simulink model "EVX_Lap_Simulation"  (R2018b)
settings: Solver=FixedStepAuto  StartTime=0  StopTime=100  FixedStep=0.01  MinStep=0.001  RelTol=1e-3
undefined symbols (not defined in the file): Car, dist, DOD, initial_velocity, motorefficiency, motormaxtorque, motorspeedradps, R0model, theta_d, Track_Dist, velocity_dnew, VoltageDOD, x, y
libraries: simulink x4
(part 3 of 3)

== matlab function EVX_Lap_Simulation/EVX Vehicle Model/Vertical Dynamics/MATLAB Function3 ==
  data: V output; F input; zB input; D output; w input; kc input; kt input; ks input; kr input
function [V,D] = Initial_SS(F,zB,w,kc,kt,ks,kr)

% syms z_WFL z_WFR z_WRL z_WRR z_c thetay thetax_F thetax_R
% 
% eq_FL = F(1) + zB(1) * kt(1)...
% 	== z_WFL * (kt(1) + ks(1) + kr(1) + kr(3) + kr(5))...
% 	 + z_WFR * (-kr(1))...
%      + z_WRL * (-kr(2))...
%      + z_wRR * (-kr(5))...
%      + z_c * (-ks(1))...
%      + thetay * (w(1,1) * ks(1))...
%      + thetax_F * (-w(2,1) * ks(1))...
%      + thetax_R * (0);
%  
% eq_FR = F(2) + zB(2) * kt(2)...
% 	== z_WFL * (-kr(1))...
% 	 + z_WFR * (kt(2) + ks(2) + kr(1) + kr(4) + kr(6))...
%      + z_WRL * (-kr(6))...
%      + z_wRR * (-kr(4))...
%      + z_c * (-ks(2))...
%      + thetay * (w(1,2) * ks(2))...
%      + thetax_F * (-w(2,2) * ks(2))...
%      + thetax_R * (0);
% 
% eq_RL = F(3) + zB(3) * kt(3)...
% 	== z_WFL * (-kr(3))...
% 	 + z_WFR * (-kr(6))...
%      + z_WRL * (kt(3) + ks(3) + kr(2) + kr(3) + kr(6))...
%      + z_wRR * (-kr(2))...
%      + z_c * (-ks(3))...
%      + thetay * (w(1,3) * ks(3))...
%      + thetax_F * (0)...
%      + thetax_R * (-w(2,3) * ks(3));
%  
% eq_RR = F(4) + zB(4) * kt(4)...
% 	== z_WFL * (-kr(5))...
% 	 + z_WFR * (-kr(4))...
%      + z_WRL * (-kr(2))...
%      + z_wRR * (kt(4) + ks(4) + kr(2) + kr(4) + kr(5))...
%      + z_c * (-ks(4))...
%      + thetay * (w(1,4) * ks(4))...
%      + thetax_F * (0)...
%      + thetax_R * (-w(2,4) * ks(4));
%  
% eq_zc = F(5)...
%     == z_WFL * (-ks(1))...
%      + z_WFR * (-ks(2))...
%      + z_WRL * (-ks(3))...
%      + z_WRR * (-ks(4))...
%      + z_c * (ks(1) + ks(2) + ks(3) + ks(4))...
%      + thetay * (-W(1,1) * ks(1) - w(1,2) * ks(2) - w(1,3) * ks(3) - w(1,4) * ks(4))...
%      + thetax_F * (w(2,1) * ks(1) + w(2,2) * ks(2))...
%      + thetax_R * (w(2,3) * ks(3) + w(2,4) * ks(4));
%  
% eq_thetay = F(6)...
%     == z_WFL * (w(1,1) * ks(1))...
%      + z_WFR * (w(1,2) * ks(2))...
%      + z_WRL * (w(1,3) * ks(3))...
%      + z_WRR * (w(1,4) * ks(4))...
%      + z_c * (-w(1,1) * ks(1) - w(1,2) * ks(2) - w(1,3) * ks(3) - w(1,4) * ks(4))...
%      + thetay * ((w(1,1))^2 * ks(1) + (w(1,2))^2 * ks(2) + (w(1,3))^2 * ks(3) + (w(1,4))^2 * ks(4))...
%      + thetax_F * (-w(1,1) * w(2,1) * ks(1) - w(1,2) * w(2,2) * ks(2))...
%      + thetax_R * (-w(1,3) * w(2,3) * ks(3) - w(1,4) * w(2,4) * ks(4));
%  
% eq_thetax_F = F(7)...
%     == z_WFL * (-w(2,1) * ks(1))...
%      + z_WFR * (-w(2,2) * ks(2))...
%      + z_WRL * (0)...
%      + z_WRR * (0)...
%      + z_c * (w(2,1) * ks(1) + w(2,2) * ks(2))...
%      + thetay * (-w(1,1) * w(2,1) * ks(1) - w(1,2) * w(2,2) * ks(2))...
%      + thetax_F * ((w(2,1))^2 * ks(1) + (w(2,2))^2 * ks(2) + kc(1))...
%      + thetax_R * (-kc(1));
% 
% eq_thetax_R = F(8)...
%     == z_WFL * (0)...
%      + z_WFR * (0)...
%      + z_WRL * (-w(2,3) * ks(3))...
%      + z_WRR * (-w(2,4) * ks(4))...
%      + z_c * (w(2,3) * ks(3) + w(2,4) * ks(4))...
%      + thetay * (-w(1,3) * w(2,3) * ks(3) - w(1,4) * w(2,4) * ks(4))...
%      + thetax_F * (-kc(1))...
%      + thetax_R * ((w(2,3))^2 * ks(3) + (w(2,4))^2 * ks(4) + kc(1));
%  
% [F,k] = equationsToMatrix([eq_FL,eq_FR,eq_RL,eq_RR,eq_zc,eq_thetay,eq_thetax_F,eq_thetax_R]);

% Force = [F(1) + zB(1) * kt(1);F(2) + zB(2) * kt(2);F(3) + zB(3) * kt(3);...
%     F(4) + zB(4) * kt(4);F(5);F(6);F(7);F(8)];

k1 = [(kt(1) + ks(1) + kr(1) + kr(3) + kr(5)),...
	 (-kr(1)),...
     (-kr(3)),...
     (-kr(5)),...
     (-ks(1)),...
     (w(1,1) * ks(1)),...
     (-w(2,1) * ks(1)),...
     (0)];
 
k2 = [(-kr(1)),...
	 (kt(2) + ks(2) + kr(1) + kr(4) + kr(6)),...
     (-kr(6)),...
     (-kr(4)),...
     (-ks(2)),...
     (w(1,2) * ks(2)),...
     (-w(2,2) * ks(2)),...
     (0)];

k3 = [(-kr(3)),...
	 (-kr(6)),...
     (kt(3) + ks(3) + kr(2) + kr(3) + kr(6)),...
     (-kr(2)),...
     (-ks(3)),...
     (w(1,3) * ks(3)),...
     (0),...
     (-w(2,3) * ks(3))];
 
k4 = [(-kr(5)),...
	 (-kr(4)),...
     (-kr(2)),...
     (kt(4) + ks(4) + kr(2) + kr(4) + kr(5)),...
     (-ks(4)),...
     (w(1,4) * ks(4)),...
     (0),...
     (-w(2,4) * ks(4))];
 
k5 = [(-ks(1)),...
     (-ks(2)),...
     (-ks(3)),...
     (-ks(4)),...
     (ks(1) + ks(2) + ks(3) + ks(4)),...
     (-w(1,1) * ks(1) - w(1,2) * ks(2) - w(1,3) * ks(3) - w(1,4) * ks(4)),...
     (w(2,1) * ks(1) + w(2,2) * ks(2)),...
     (w(2,3) * ks(3) + w(2,4) * ks(4))];
 
k6 = [(w(1,1) * ks(1)),...
     (w(1,2) * ks(2)),...
     (w(1,3) * ks(3)),...
     (w(1,4) * ks(4)),...
     (-w(1,1) * ks(1) - w(1,2) * ks(2) - w(1,3) * ks(3) - w(1,4) * ks(4)),...
     ((w(1,1))^2 * ks(1) + (w(1,2))^2 * ks(2) + (w(1,3))^2 * ks(3) + (w(1,4))^2 * ks(4)),...
     (-w(1,1) * w(2,1) * ks(1) - w(1,2) * w(2,2) * ks(2)),...
     (-w(1,3) * w(2,3) * ks(3) - w(1,4) * w(2,4) * ks(4))];
 
k7 = [(-w(2,1) * ks(1)),...
     (-w(2,2) * ks(2)),...
     (0),...
     (0),...
     (w(2,1) * ks(1) + w(2,2) * ks(2)),...
     (-w(1,1) * w(2,1) * ks(1) - w(1,2) * w(2,2) * ks(2)),...
     ((w(2,1))^2 * ks(1) + (w(2,2))^2 * ks(2) + kc(1)),...
     (-kc(1))];

k8 = [(0),...
     (0),...
     (-w(2,3) * ks(3)),...
     (-w(2,4) * ks(4)),...
     (w(2,3) * ks(3) + w(2,4) * ks(4)),...
     (-w(1,3) * w(2,3) * ks(3) - w(1,4) * w(2,4) * ks(4)),...
     (-kc(1)),...
     ((w(2,3))^2 * ks(3) + (w(2,4))^2 * ks(4) + kc(1))];

% D = linsolve(F,k);

k = [k1;k2;k3;k4;k5;k6;k7;k8];

D = (F/k)';

V = [0;0;0;0;0;0;0;0];

== matlab function EVX_Lap_Simulation/EVX Vehicle Model/Vertical Dynamics/MATLAB Function5 ==
  data: D input; F_T output; V input; kt input; ct input
function F_T  = Tyre_Forces(D,V,kt,ct)

D = D(1:4,:);
V = V(1:4,:);

F_T = D .* kt + V .* ct;

F_T(F_T > 0) = 0;

== matlab function EVX_Lap_Simulation/EVX Vehicle Model/Wheel Dynamics/Wheel Acceleration ==
  data: F_x input; T input; I input; ddwheel output; r input
function ddwheel   = Wheel_Acceleration(F_x,T,I,r)


ddwheel = (T - (F_x .* r))./I;
